simulink model "vander3d"  (R2023a)
settings: Solver=ode1  StartTime=0.0  StopTime=500  FixedStep=0.002  RelTol=1e-3
values from neighbouring files (symbols this model uses):
  beta3d = 0.9    [loadResultData.m]    (also in simulate_hover.m; temp.m)
  cycleGain = 0.2    [simulate_hover.m]    (also in temp.m = 1)
  epsilon3d = 1    [loadResultData.m]    (also in simulate_hover.m; temp.m)
  k3d = 1.65    [loadResultData.m]    (also in simulate_hover.m; temp.m)
settings Model: Creator=Jacob  LastModifiedBy=Jacob
settings DataIOCC: ReturnWorkspaceOutputs=off

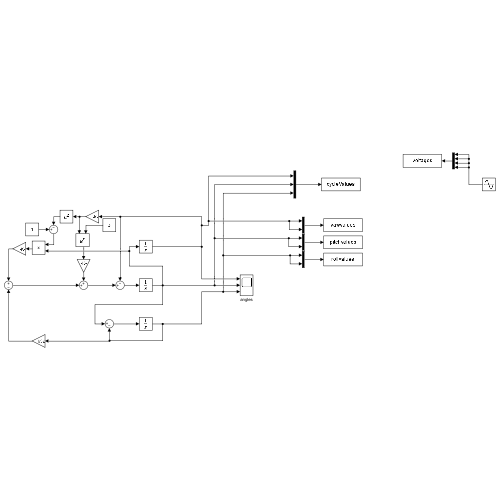
[thumbnail: Simulink's stored preview of the top-level diagram]
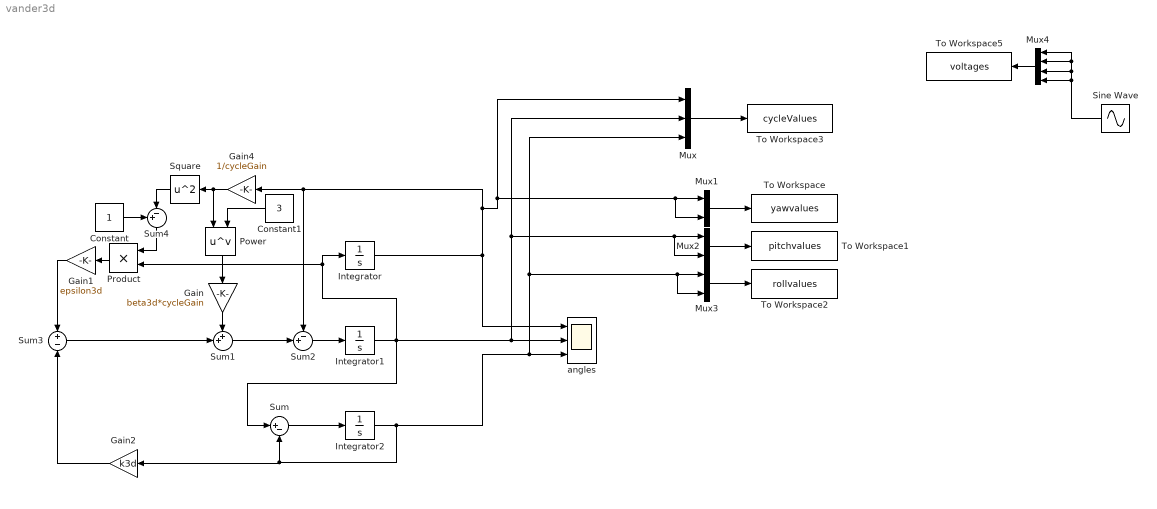
== system vander3d ==
  Constant : Constant
  Constant1 : Constant  Value=3
  Gain : Gain  Gain=beta3d*cycleGain
  Gain1 : Gain  Gain=epsilon3d
  Gain2 : Gain  Gain=k3d
  Gain4 : Gain  Gain=1/cycleGain
  Integrator : Integrator  InitialCondition=0.0001
  Integrator1 : Integrator  InitialCondition=0.0001
  Integrator2 : Integrator  InitialCondition=0.0001
  Mux : Mux  Inputs=3
  Mux1 : Mux  Inputs=2
  Mux2 : Mux  Inputs=2
  Mux3 : Mux  Inputs=2
  Mux4 : Mux
  Power : Math  Operator=pow
  Product : Product
  Sine Wave : Sin  SampleTime=0
  Square : Math  Operator=square
  Sum : Sum  Inputs=|+-
  Sum1 : Sum  Inputs=++|
  Sum2 : Sum  Inputs=-+|
  Sum3 : Sum  Inputs=+|-
  Sum4 : Sum  Inputs=+-|
  To Workspace : ToWorkspace  VariableName=yawvalues  SampleTime=-1
  To Workspace1 : ToWorkspace  VariableName=pitchvalues  SampleTime=-1
  To Workspace2 : ToWorkspace  VariableName=rollvalues  SampleTime=-1
  To Workspace3 : ToWorkspace  VariableName=cycleValues  SampleTime=-1
  To Workspace5 : ToWorkspace  VariableName=voltages  SampleTime=-1
  angles : Scope  NumInputPorts=3
  wires:
  Integrator1/1 -> Sum/1, Mux2/2, Mux2/1, Mux/2, angles/2, Product/2, Integrator/1
  Sum/1 -> Integrator2/1
  Integrator2/1 -> Mux3/2, Mux3/1, Mux/3, angles/3, Sum/2, Gain2/1
  Sum1/1 -> Sum2/2
  Sum2/1 -> Integrator1/1
  Constant1/1 -> Power/2
  Power/1 -> Gain/1
  Gain/1 -> Sum1/1
  Sum3/1 -> Sum1/2
  Sum4/1 -> Product/1
  Product/1 -> Gain1/1
  Gain1/1 -> Sum3/1
  Constant/1 -> Sum4/1
  Square/1 -> Sum4/2
  Gain2/1 -> Sum3/2
  Integrator/1 -> angles/1, Sum2/1, Gain4/1, Mux1/2, Mux1/1, Mux/1
  Gain4/1 -> Square/1, Power/1
  Mux/1 -> To Workspace3/1
  Mux4/1 -> To Workspace5/1
  Sine Wave/1 -> Mux4/4, Mux4/3, Mux4/2, Mux4/1
  Mux3/1 -> To Workspace2/1
  Mux1/1 -> To Workspace/1
  Mux2/1 -> To Workspace1/1
